simulink model "Sim_V_in"  (R2024b)
settings: Solver=VariableStepAuto  StartTime=0.0  StopTime=sim.t  RelTol=1e-3
values from neighbouring files (symbols this model uses):
  B = [-sqrt(6).*Kt/(3.*Rm.*(Iy-Iw)) sqrt(6).*Kt/(6.*Rm.*(Iy-Iw)) sqrt(6).*Kt/(6.*Rm.*(Iy-Iw)) ;0 -sqrt(2).*Kt/(2.*Rm.*(Ix-Iw)) sqrt(2).*Kt/(2.*Rm.*(Ix-Iw)) ; -sqrt(3).*Kt/(3.*Rm.*(Iz-Iw)) -sqrt(3).*Kt/(3.*Rm.*(Iz-Iw)) -sqrt(3).*Kt/(3.*Rm.*(Iz-Iw));0 0 0;0 0 0;Kt/(Rm.*Iw) 0 0;0 Kt/(Rm.*Iw) 0;0 0 Kt/(Rm.*Iw)]    [test.m]
undefined symbols (not defined in the file or in its folder): cube, cube_acc, d_theta, Earth, h, motor, ref, rw_acc, sim, vin, WGS84
libraries: slpidlib x3, aerolibfltsims x2, aerolibsim3d x2, aerolibtransform2 x1, aerolibanim x1, sim3dlib x1
settings Model: Creator=ben  LastModifiedBy=ben

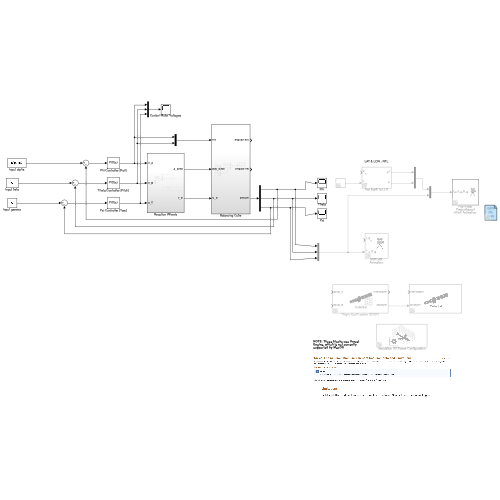
[thumbnail: Simulink's stored preview of the top-level diagram]
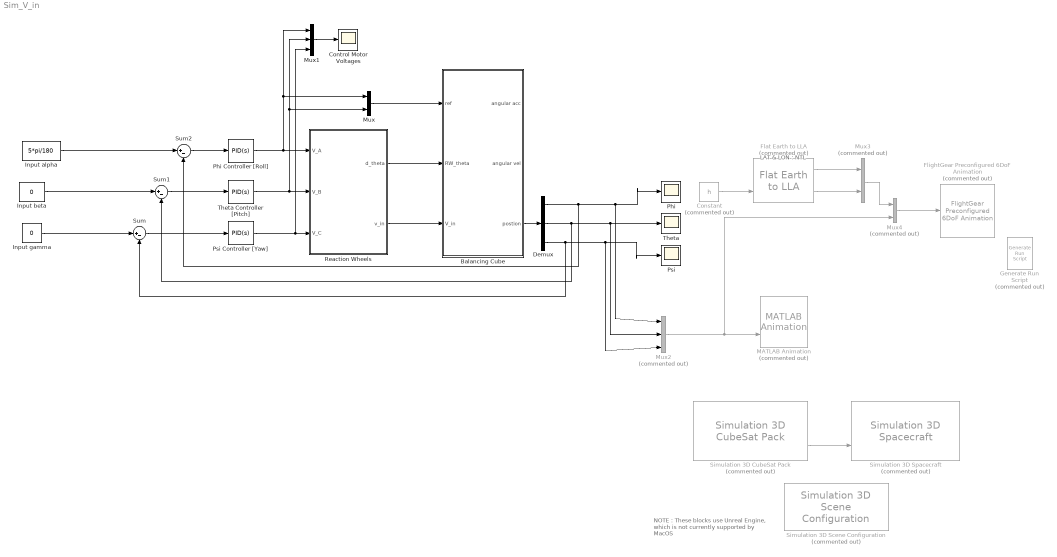
== system Sim_V_in ==
  note: LAT & LON : NTL
  note: NOTE : These blocks use Unreal Engine, which is not currently supported by MacOS
  Balancing Cube : Subsystem
  Constant : Constant  Commented=on  Value=h
  Control Motor Voltages : Scope
  Demux : Demux  Outputs=3
  Flat Earth to LLA : aerolibtransform2/Flat Earth to LLA  Commented=on  units=Metric (MKS)  ptype=Earth (WGS84)  F=1/298.257223563  R=6378137  refPosPort=off  LL0=[22 150]  psi=0
  FlightGear Preconfigured 6DoF Animation : aerolibfltsims/FlightGear Preconfigured 6DoF Animation  Commented=on  xFlightGearVersion=v2019.1  DestinationIpAddress=127.0.0.1  DestinationPort=5502  SampleTime=1/20  packetVersion=24
  Generate Run Script : aerolibfltsims/Generate Run Script  Commented=on  Architecture=Mac  dataFlow=Send  GeometryModelName=c172p  AirportId=YSSY  RunwayId=10L  InitialAltitude=7224  InitialHeading=113  OffsetDistance=4.72  OffsetAzimuth=0  InstallScenery=on  DisableShaders=on  OriginAddress=127.0.0.1  DestinationPort=5502  OriginPort=5505  LocalAddress=127.0.0.1  OutputFileName=runfg2.sh  FlightGearBaseDirectory=/Applications/FlightGear.app
  Input alpha : Constant  Value=5*pi/180  SampleTime=0.1
  Input beta : Constant  Value=0  SampleTime=0.1
  Input gamma : Constant  Value=0  SampleTime=0.1
  MATLAB Animation : aerolibanim/MATLAB Animation  Tag=Matlab Animation 6 DOF  Commented=on  Vehicles=1  Geometries='pa24-250_orange.ac'  BoundingBoxCoordinates=[-50,50,-50,50,-50,50]  CameraOffset=[-150,0,0]  CameraViewAngle=5  SampleTime=0.01  FigurePosition=[761,102,744,779]
  Mux : Mux  Inputs=2
  Mux1 : Mux  Inputs=3
  Mux2 : Mux  Commented=on  Inputs=3
  Mux3 : Mux  Commented=on  Inputs=2
  Mux4 : Mux  Commented=on  Inputs=2
  Phi : Scope
  Phi Controller [Roll] : slpidlib/PID Controller  Controller=PID  Form=Parallel  TimeDomain=Continuous-time  UseExternalTs=off  SampleTime=-1  IntegratorMethod=Forward Euler  FilterMethod=Forward Euler  ControllerParametersSource=internal  P=-50.4825434106595  I=-1.23008759816909  UseKiTs=off  D=-412.023535687071  UseExternalDerivativeSource=off  N=0.379397383172155  UseFilter=on  TunerSelectOption=Transfer Function Based (PID Tuner App)  InitialConditionSource=internal  InitialConditionForIntegrator=0  InitialConditionForFilter=0  DifferentiatorICPrevScaledInput=0  ExternalReset=none  TrackingMode=off  Kt=1  LimitOutput=off  SatLimitsSource=internal  UpperSaturationLimit=inf  LowerSaturationLimit=-inf  LinearizeAsGain=on  AntiWindupMode=none  Kb=1  LimitIntegrator=off  UpperIntegratorSaturationLimit=inf  LowerIntegratorSaturationLimit=-inf  POutMin=[]  POutMax=[]  IOutMin=[]  IOutMax=[]  DOutMin=[]  DOutMax=[]  NOutMin=[]  NOutMax=[]  SumOutMin=[]  SumOutMax=[]  SaturationOutMin=[]  SaturationOutMax=[]  PParamMin=[]  PParamMax=[]  IParamMin=[]  IParamMax=[]  DParamMin=[]  DParamMax=[]  NParamMin=[]  NParamMax=[]  KbParamMin=[]  KbParamMax=[]  KtParamMin=[]  KtParamMax=[]  KbOutMin=[]  KbOutMax=[]  KtOutMin=[]  KtOutMax=[]  IntegratorOutMin=[]  IntegratorOutMax=[]  FilterOutMin=[]  FilterOutMax=[]  SumI1OutMin=[]  SumI1OutMax=[]  SumI2OutMin=[]  SumI2OutMax=[]  SumI3OutMin=[]  SumI3OutMax=[]  SumI4OutMin=[]  SumI4OutMax=[]  SumDOutMin=[]  SumDOutMax=[]  DifferentiatorOutMin=[]  DifferentiatorOutMax=[]  FilterDiffOutCoefMin=[]  FilterDiffOutCoefMax=[]  ReciprocalOutMin=[]  ReciprocalOutMax=[]  SumDenOutMin=[]  SumDenOutMax=[]  SumNumOutMin=[]  SumNumOutMax=[]  DivideOutMin=[]  DivideOutMax=[]  UdiffTsProdOutMin=[]  UdiffTsProdOutMax=[]  NTsProdOutMin=[]  NTsProdOutMax=[]  UintegralTsProdOutMin=[]  UintegralTsProdOutMax=[]  UngainTsProdOutMin=[]  UngainTsProdOutMax=[]  ClampingZeroOutDataTypeStr=Inherit: Inherit via back propagation  ClampingZeroOutMin=[]  ClampingZeroOutMax=[]  FilterDenConstantOutDataTypeStr=Inherit: Inherit via back propagation  FilterDenConstantOutMin=[]  FilterDenConstantOutMax=[]  PCopyOutDataTypeStr=Inherit: Inherit via back propagation  PCopyOutMin=[]  PCopyOutMax=[]  NCopyOutDataTypeStr=Inherit: Inherit via back propagation  NCopyOutMin=[]  NCopyOutMax=[]  IntegratorContinuousStateAttributes=''  IntegratorStateMustResolveToSignalObject=off  IntegratorRTWStateStorageClass=Auto  FilterContinuousStateAttributes=''  FilterStateMustResolveToSignalObject=off  FilterRTWStateStorageClass=Auto  ParallelPVariant=InternalParameters  IdealPVariant=Disabled  IVariant=InternalParameters  DVariant=InternalParameters  IntegratorVariant=Continuous  SatVariant=Disabled  AWVariant=Passthrough  PCopyVariant=Disabled  TRVariant=Disabled  FdbkBlocksVariant=Forward  IdealPFdbkVariant=Disabled  SatFdbkVariant=Disabled  DerivativeFilterVariant=ContFilter  NVariant=InternalParameters  NCopyVariant=Disabled  FilterICVariant=InternalICsFilter  IntegratorICVariant=InternalICs  ExternalResetVariant=Disabled  TRSumVariant=Passthrough  SumFdbkVariant=Disabled  SumVariant=Sum_PID  TsampFilterVariant=InternalTs  TsampNgainVariant=Passthrough  TsampIntegralVariant=Disabled_SignalSpec  ExternalSaturationOutDataTypeStr=Inherit: Same as second input  DerivativeSourceVariant=ErrorSignal  PreIntVariant=InternalPreInt
  Psi : Scope
  Psi Controller [Yaw] : slpidlib/PID Controller  Controller=PID  Form=Parallel  TimeDomain=Continuous-time  UseExternalTs=off  SampleTime=-1  IntegratorMethod=Forward Euler  FilterMethod=Forward Euler  ControllerParametersSource=internal  P=-763.325878025154  I=-72.3330718489805  UseKiTs=off  D=-1552.13165448844  UseExternalDerivativeSource=off  N=226.089930864036  UseFilter=on  TunerSelectOption=Transfer Function Based (PID Tuner App)  InitialConditionSource=internal  InitialConditionForIntegrator=0  InitialConditionForFilter=0  DifferentiatorICPrevScaledInput=0  ExternalReset=none  TrackingMode=off  Kt=1  LimitOutput=off  SatLimitsSource=internal  UpperSaturationLimit=inf  LowerSaturationLimit=-inf  LinearizeAsGain=on  AntiWindupMode=none  Kb=1  LimitIntegrator=off  UpperIntegratorSaturationLimit=inf  LowerIntegratorSaturationLimit=-inf  POutMin=[]  POutMax=[]  IOutMin=[]  IOutMax=[]  DOutMin=[]  DOutMax=[]  NOutMin=[]  NOutMax=[]  SumOutMin=[]  SumOutMax=[]  SaturationOutMin=[]  SaturationOutMax=[]  PParamMin=[]  PParamMax=[]  IParamMin=[]  IParamMax=[]  DParamMin=[]  DParamMax=[]  NParamMin=[]  NParamMax=[]  KbParamMin=[]  KbParamMax=[]  KtParamMin=[]  KtParamMax=[]  KbOutMin=[]  KbOutMax=[]  KtOutMin=[]  KtOutMax=[]  IntegratorOutMin=[]  IntegratorOutMax=[]  FilterOutMin=[]  FilterOutMax=[]  SumI1OutMin=[]  SumI1OutMax=[]  SumI2OutMin=[]  SumI2OutMax=[]  SumI3OutMin=[]  SumI3OutMax=[]  SumI4OutMin=[]  SumI4OutMax=[]  SumDOutMin=[]  SumDOutMax=[]  DifferentiatorOutMin=[]  DifferentiatorOutMax=[]  FilterDiffOutCoefMin=[]  FilterDiffOutCoefMax=[]  ReciprocalOutMin=[]  ReciprocalOutMax=[]  SumDenOutMin=[]  SumDenOutMax=[]  SumNumOutMin=[]  SumNumOutMax=[]  DivideOutMin=[]  DivideOutMax=[]  UdiffTsProdOutMin=[]  UdiffTsProdOutMax=[]  NTsProdOutMin=[]  NTsProdOutMax=[]  UintegralTsProdOutMin=[]  UintegralTsProdOutMax=[]  UngainTsProdOutMin=[]  UngainTsProdOutMax=[]  ClampingZeroOutDataTypeStr=Inherit: Inherit via back propagation  ClampingZeroOutMin=[]  ClampingZeroOutMax=[]  FilterDenConstantOutDataTypeStr=Inherit: Inherit via back propagation  FilterDenConstantOutMin=[]  FilterDenConstantOutMax=[]  PCopyOutDataTypeStr=Inherit: Inherit via back propagation  PCopyOutMin=[]  PCopyOutMax=[]  NCopyOutDataTypeStr=Inherit: Inherit via back propagation  NCopyOutMin=[]  NCopyOutMax=[]  IntegratorContinuousStateAttributes=''  IntegratorStateMustResolveToSignalObject=off  IntegratorRTWStateStorageClass=Auto  FilterContinuousStateAttributes=''  FilterStateMustResolveToSignalObject=off  FilterRTWStateStorageClass=Auto  ParallelPVariant=InternalParameters  IdealPVariant=Disabled  IVariant=InternalParameters  DVariant=InternalParameters  IntegratorVariant=Continuous  SatVariant=Disabled  AWVariant=Passthrough  PCopyVariant=Disabled  TRVariant=Disabled  FdbkBlocksVariant=Forward  IdealPFdbkVariant=Disabled  SatFdbkVariant=Disabled  DerivativeFilterVariant=ContFilter  NVariant=InternalParameters  NCopyVariant=Disabled  FilterICVariant=InternalICsFilter  IntegratorICVariant=InternalICs  ExternalResetVariant=Disabled  TRSumVariant=Passthrough  SumFdbkVariant=Disabled  SumVariant=Sum_PID  TsampFilterVariant=InternalTs  TsampNgainVariant=Passthrough  TsampIntegralVariant=Disabled_SignalSpec  ExternalSaturationOutDataTypeStr=Inherit: Same as second input  DerivativeSourceVariant=ErrorSignal  PreIntVariant=InternalPreInt
  Reaction Wheels : Subsystem
  Simulation 3D CubeSat Pack : aerolibsim3d/Simulation 3D CubeSat Pack  Commented=on  Antenna1_T=off  Antenna1_R=off  Antenna2_T=off  Antenna2_R=off  Antenna3_T=off  Antenna3_R=off  Sensor_T=off  Sensor_R=off  SolarArray1_T=off  SolarArray1_R=off  SolarArray1_1_T=off  SolarArray1_1_R=off  SolarArray2_T=off  SolarArray2_R=off  SolarArray2_2_T=off  SolarArray2_2_R=off  Thruster_T=off  Thruster_R=off  GeoRadioButton=ECEF  AdjustForCesium=on  Heading0=90
      settings: AttributesFormatString=Origin: Earth center (ECEF)
  Simulation 3D Scene Configuration : sim3dlib/Simulation 3D Scene Configuration  Priority=0  Commented=on  ProjectFormat=Default Scenes  SceneDesc=Airport  ProjectName=B:\matlab\toolbox\shared\sim3d_projects\automotive_project_windows\UE\WindowsNoEditor\VehicleSimulation.exe  ScenePath=/Game/Maps/HwStrght  EnableOpenDRIVE=off  vehTagList={'Custom';'Scene Origin';'SimulinkVehicle1'}  vehTag=Scene Origin  FreeCameraInitialTranslation=[-6, 0, 2]  FreeCameraDefaultInitialTranslation=[-6, 0, 2]  FreeCameraInitialRotation=[0, -15, 0]  FreeCameraDefaultInitialRotation=[0, -15, 0]  OpVisEn=off  Ts=.02  EnableWindow=on  EnableRemoteAccess=off  EnableWeather=off  SunAzimuth=90  SunAltitude=40.0  EnableGeospatialSun=off  Latitude=0  Longitude=0  Date=2023-01-01  Time=10:30:00  GeoTimeZone=-5.0  SunDaylightSaving=off  wind=1  clouds=10  EnableVolumetricClouds=off  CloudCoverage=0  CloudAltitude=6  fog=0  rain=0  RaindropsEffect=off  SnowDensity=0  EnableGeospatial=off  UseTrueOrigin=off  OriginHeight=200  OriginLatitude=40.744652  OriginLongitude=-73.988864  MapStyle=Aerial  AdditionalAssetIDs=[]  UseAdvancedSunSky=off  SolarTime=11  TimeZone=-5  Day=21  Month=9  Year=2022  UseDaylightSavingTime=on  DSTStartDay=10  DSTStartMonth=3  DSTEndDay=3  DSTEndMonth=11  DSTSwitchHour=2  sensorTag=MainCamera1  sensorId=1  sensorName=MainCamera1  mountLoc=Origin  offsetFlag=off  tmountOffset=[0, 0, 0]  rmountOffset=[0, 0, 0]  HorizontalResolution=1280  VerticalResolution=720  HorizontalFOV=60  mountPoint=[0 0 0]  mountOrientation=[0 0 0]  aMode=0  ID=1  GeoTrigger=Inactive
      settings: LibrarySourceBlock=aerolibsim3d/Simulation 3D Scene Configuration
  Simulation 3D Spacecraft : aerolibsim3d/Simulation 3D Spacecraft  Priority=1  Commented=on  Mesh=CubeSat  MeshPath=/MathWorksAerospaceContent/Vehicles/Spacecraft/CubeSat/Mesh/SK_CubeSat.SK_CubeSat  MeshPathSmall=/MathWorksAerospaceContent/Vehicles/Spacecraft/SmallSat/Mesh/SK_SmallSat.SK_SmallSat  SpacecraftColor=Silver  ActorName=SimulinkVehicle1  Translation=zeros(10, 3)  Rotation=zeros(10, 3)  ScaleInputPort=Dialog  Scale=[1 1 1]  InitialScale=[1 1 1]  IsGHSensorEnabled=off  AreGHRaysVisible=off  IsOutputReshapeEnabled=on  GHRayLength=1524  GHBodyOffset=1  GHContactLocation1=[0 0 0]  GHContactLocation2=[0 0 0]  GHContactLocation3=[0 0 0]  GHContactLocation4=[0 0 0]  WoWSensorTolerance=0.05  SampleTime=-1  ActorType=SimulinkVehicle  ID=1  aMode=0  ActorTag=SimulinkVehicle1
  Sum : Sum  Inputs=|+-
  Sum1 : Sum  Inputs=|+-
  Sum2 : Sum  Inputs=|+-
  Theta : Scope
  Theta Controller [Pitch] : slpidlib/PID Controller  Controller=PID  Form=Parallel  TimeDomain=Continuous-time  UseExternalTs=off  SampleTime=-1  IntegratorMethod=Forward Euler  FilterMethod=Forward Euler  ControllerParametersSource=internal  P=-456.390816139374  I=-30.5631615457373  UseKiTs=off  D=-1701.86514883062  UseExternalDerivativeSource=off  N=163.363333487621  UseFilter=on  TunerSelectOption=Transfer Function Based (PID Tuner App)  InitialConditionSource=internal  InitialConditionForIntegrator=0  InitialConditionForFilter=0  DifferentiatorICPrevScaledInput=0  ExternalReset=none  TrackingMode=off  Kt=1  LimitOutput=off  SatLimitsSource=internal  UpperSaturationLimit=inf  LowerSaturationLimit=-inf  LinearizeAsGain=on  AntiWindupMode=none  Kb=1  LimitIntegrator=off  UpperIntegratorSaturationLimit=inf  LowerIntegratorSaturationLimit=-inf  POutMin=[]  POutMax=[]  IOutMin=[]  IOutMax=[]  DOutMin=[]  DOutMax=[]  NOutMin=[]  NOutMax=[]  SumOutMin=[]  SumOutMax=[]  SaturationOutMin=[]  SaturationOutMax=[]  PParamMin=[]  PParamMax=[]  IParamMin=[]  IParamMax=[]  DParamMin=[]  DParamMax=[]  NParamMin=[]  NParamMax=[]  KbParamMin=[]  KbParamMax=[]  KtParamMin=[]  KtParamMax=[]  KbOutMin=[]  KbOutMax=[]  KtOutMin=[]  KtOutMax=[]  IntegratorOutMin=[]  IntegratorOutMax=[]  FilterOutMin=[]  FilterOutMax=[]  SumI1OutMin=[]  SumI1OutMax=[]  SumI2OutMin=[]  SumI2OutMax=[]  SumI3OutMin=[]  SumI3OutMax=[]  SumI4OutMin=[]  SumI4OutMax=[]  SumDOutMin=[]  SumDOutMax=[]  DifferentiatorOutMin=[]  DifferentiatorOutMax=[]  FilterDiffOutCoefMin=[]  FilterDiffOutCoefMax=[]  ReciprocalOutMin=[]  ReciprocalOutMax=[]  SumDenOutMin=[]  SumDenOutMax=[]  SumNumOutMin=[]  SumNumOutMax=[]  DivideOutMin=[]  DivideOutMax=[]  UdiffTsProdOutMin=[]  UdiffTsProdOutMax=[]  NTsProdOutMin=[]  NTsProdOutMax=[]  UintegralTsProdOutMin=[]  UintegralTsProdOutMax=[]  UngainTsProdOutMin=[]  UngainTsProdOutMax=[]  ClampingZeroOutDataTypeStr=Inherit: Inherit via back propagation  ClampingZeroOutMin=[]  ClampingZeroOutMax=[]  FilterDenConstantOutDataTypeStr=Inherit: Inherit via back propagation  FilterDenConstantOutMin=[]  FilterDenConstantOutMax=[]  PCopyOutDataTypeStr=Inherit: Inherit via back propagation  PCopyOutMin=[]  PCopyOutMax=[]  NCopyOutDataTypeStr=Inherit: Inherit via back propagation  NCopyOutMin=[]  NCopyOutMax=[]  IntegratorContinuousStateAttributes=''  IntegratorStateMustResolveToSignalObject=off  IntegratorRTWStateStorageClass=Auto  FilterContinuousStateAttributes=''  FilterStateMustResolveToSignalObject=off  FilterRTWStateStorageClass=Auto  ParallelPVariant=InternalParameters  IdealPVariant=Disabled  IVariant=InternalParameters  DVariant=InternalParameters  IntegratorVariant=Continuous  SatVariant=Disabled  AWVariant=Passthrough  PCopyVariant=Disabled  TRVariant=Disabled  FdbkBlocksVariant=Forward  IdealPFdbkVariant=Disabled  SatFdbkVariant=Disabled  DerivativeFilterVariant=ContFilter  NVariant=InternalParameters  NCopyVariant=Disabled  FilterICVariant=InternalICsFilter  IntegratorICVariant=InternalICs  ExternalResetVariant=Disabled  TRSumVariant=Passthrough  SumFdbkVariant=Disabled  SumVariant=Sum_PID  TsampFilterVariant=InternalTs  TsampNgainVariant=Passthrough  TsampIntegralVariant=Disabled_SignalSpec  ExternalSaturationOutDataTypeStr=Inherit: Same as second input  DerivativeSourceVariant=ErrorSignal  PreIntVariant=InternalPreInt
  wires:
  Phi Controller [Roll]/1 -> Mux/1, Mux1/1, Reaction Wheels/1(V_A)
  Psi Controller [Yaw]/1 -> Reaction Wheels/3(V_C), Mux1/3
  Theta Controller [Pitch]/1 -> Reaction Wheels/2(V_B), Mux/2, Mux1/2
  Sum2/1 -> Phi Controller [Roll]/1
  Sum1/1 -> Theta Controller [Pitch]/1
  Sum/1 -> Psi Controller [Yaw]/1
  Demux/1 -> Sum2/2, Mux2/1, Phi/1
  Demux/2 -> Mux2/2, Theta/1, Sum1/2
  Demux/3 -> Sum/2, Mux2/3, Psi/1
  Mux1/1 -> Control Motor Voltages/1
  Simulation 3D CubeSat Pack/2 -> Simulation 3D Spacecraft/2
  Mux4/1 -> FlightGear Preconfigured 6DoF Animation/1
  Mux3/1 -> Mux4/1
  Mux2/1 -> MATLAB Animation/2, Mux4/2
  Flat Earth to LLA/2 -> Mux3/2
  Constant/1 -> Flat Earth to LLA/2
  Flat Earth to LLA/1 -> Mux3/1
  Input alpha/1 -> Sum2/1
  Input beta/1 -> Sum1/1
  Input gamma/1 -> Sum/1
  Reaction Wheels/1(d_theta) -> Balancing Cube/2(RW_theta)
  Reaction Wheels/2(v_in) -> Balancing Cube/3(V_in)
  Mux/1 -> Balancing Cube/1(ref)
  Balancing Cube/3(postion) -> Demux/1

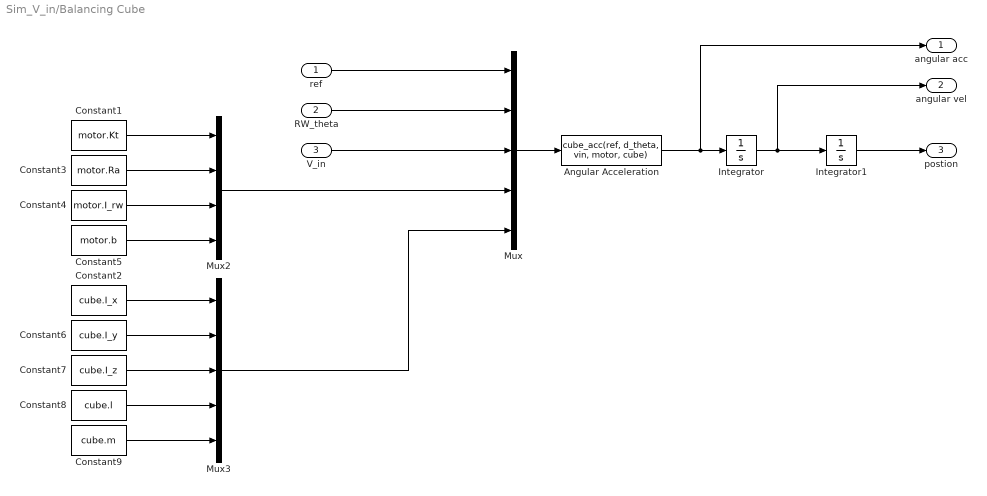
== system Sim_V_in/Balancing Cube ==
  ref : Inport
  RW_theta : Inport  Port=2
  V_in : Inport  Port=3
  Angular Acceleration : MATLABFcn  MATLABFcn=cube_acc(ref, d_theta, vin, motor, cube)
  Constant1 : Constant  Value=motor.Kt
  Constant2 : Constant  Value=cube.I_x
  Constant3 : Constant  Value=motor.Ra
  Constant4 : Constant  Value=motor.I_rw
  Constant5 : Constant  Value=motor.b
  Constant6 : Constant  Value=cube.I_y
  Constant7 : Constant  Value=cube.I_z
  Constant8 : Constant  Value=cube.l
  Constant9 : Constant  Value=cube.m
  Integrator : Integrator  InitialCondition=sim.cube_ic_vel
  Integrator1 : Integrator  InitialCondition=sim.cube_ic_pos
  Mux : Mux  Inputs=5
  Mux2 : Mux
  Mux3 : Mux  Inputs=5
  angular acc : Outport
  angular vel : Outport  Port=2
  postion : Outport  Port=3
  wires:
  Mux/1 -> Angular Acceleration/1
  Angular Acceleration/1 -> angular acc/1, Integrator/1
  Integrator/1 -> Integrator1/1, angular vel/1
  ref/1 -> Mux/1
  RW_theta/1 -> Mux/2
  V_in/1 -> Mux/3
  Integrator1/1 -> postion/1
  Constant5/1 -> Mux2/4
  Constant3/1 -> Mux2/2
  Constant4/1 -> Mux2/3
  Constant9/1 -> Mux3/5
  Constant7/1 -> Mux3/3
  Constant1/1 -> Mux2/1
  Constant6/1 -> Mux3/2
  Constant2/1 -> Mux3/1
  Constant8/1 -> Mux3/4
  Mux2/1 -> Mux/4
  Mux3/1 -> Mux/5

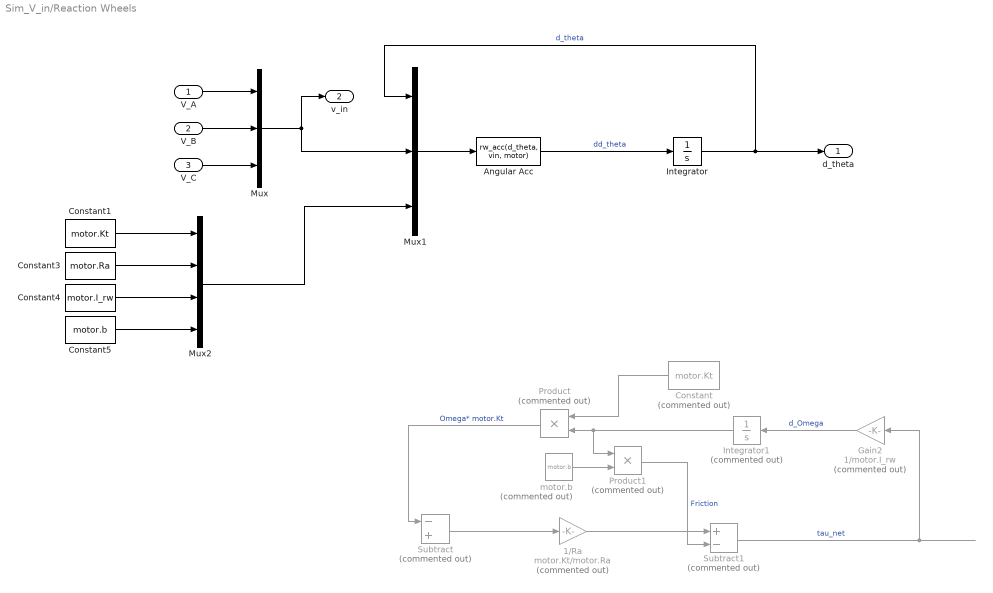
== system Sim_V_in/Reaction Wheels ==
  V_A : Inport
  V_B : Inport  Port=2
  V_C : Inport  Port=3
  1/Ra : Gain  Commented=on  Gain=motor.Kt/motor.Ra
  Angular Acc : MATLABFcn  MATLABFcn=rw_acc(d_theta, vin, motor)
  Constant : Constant  Commented=on  Value=motor.Kt
  Constant1 : Constant  Value=motor.Kt
  Constant3 : Constant  Value=motor.Ra
  Constant4 : Constant  Value=motor.I_rw
  Constant5 : Constant  Value=motor.b
  Gain2 : Gain  Commented=on  Gain=1/motor.I_rw
  Integrator : Integrator  InitialCondition=sim.rw_ic
  Integrator1 : Integrator  Commented=on
  Mux : Mux  Inputs=3
  Mux1 : Mux  Inputs=3
  Mux2 : Mux
  Product : Product  Commented=on
  Product1 : Product  Commented=on
  Subtract : Sum  Commented=on  Inputs=-+
  Subtract1 : Sum  Commented=on  Inputs=+-
  motor.b : Constant  Commented=on  Value=motor.b  VectorParams1D=off
  d_theta : Outport
  v_in : Outport  Port=2
  wires:
  Angular Acc/1 -> Integrator/1  "dd_theta"
  Integrator/1 -> Mux1/1, d_theta/1  "d_theta"
  V_A/1 -> Mux/1
  V_B/1 -> Mux/2
  V_C/1 -> Mux/3
  Subtract/1 -> 1/Ra/1
  Product/1 -> Subtract/1  "Omega* motor.Kt"
  Constant/1 -> Product/1
  1/Ra/1 -> Subtract1/1
  motor.b/1 -> Product1/2
  Gain2/1 -> Integrator1/1  "d_Omega"
  Product1/1 -> Subtract1/2  "Friction"
  Integrator1/1 -> Product1/1, Product/2
  Subtract1/1 -> Gain2/1  "tau_net"
  Mux1/1 -> Angular Acc/1
  Mux/1 -> v_in/1, Mux1/2
  Mux2/1 -> Mux1/3
  Constant1/1 -> Mux2/1
  Constant3/1 -> Mux2/2
  Constant5/1 -> Mux2/4
  Constant4/1 -> Mux2/3
